simulink model "CM640C_MotAg1Meas"  (R2013b)
settings: Solver=VariableStepDiscrete  SolverMode=SingleTasking  StartTime=0.0  StopTime=1  FixedStep=0.002  RelTol=1e-3
values from neighbouring files (symbols this model uses):
  ARCHGLBPRM_2PI_ULS_F32 = DataDict.Constant    [CM640C_MotAg1Meas_DataDict.m]
  CNTPERREV_MOTREV_S15P16 = DataDict.Constant    [CM640C_MotAg1Meas_DataDict.m]
  COEFFTBLELMSIZE_CNT_U08 = DataDict.Constant    [CM640C_MotAg1Meas_DataDict.m]
  COEFFTBLSIZE_CNT_U08 = DataDict.Constant    [CM640C_MotAg1Meas_DataDict.m]
  CORRNTBLAGSTEPSIZE_MATRAD_F32 = DataDict.Constant    [CM640C_MotAg1Meas_DataDict.m]
  CORRNTBLSIDXOFFS_CNT_U16 = DataDict.Constant    [CM640C_MotAg1Meas_DataDict.m]
  CORRNTBLSIZE_CNT_U16 = DataDict.Constant    [CM640C_MotAg1Meas_DataDict.m]
  CORRNTBLSIZEMASK_CNT_U08 = DataDict.Constant    [CM640C_MotAg1Meas_DataDict.m]
  MOTAG1ERRTHD_MOTREV_U0P16 = DataDict.Constant    [CM640C_MotAg1Meas_DataDict.m]
  MotAg1MeasMotAgOffs = DataDict.Calibration    [CM640C_MotAg1Meas_DataDict.m]
  MotAg1PrtclFlt = DataDict.NTC    [CM640C_MotAg1Meas_DataDict.m]
  MOTAG1PRTCLFLTFAILSTEP_CNT_U16 = DataDict.Constant    [CM640C_MotAg1Meas_DataDict.m]
  MOTAG1PRTCLFLTPASSSTEP_CNT_U16 = DataDict.Constant    [CM640C_MotAg1Meas_DataDict.m]
  MOTAGCPTLIMFLTMASK_CNT_U32 = DataDict.Constant    [CM640C_MotAg1Meas_DataDict.m]
  MOTAGDELTAPERCORRNPT_CNT_U16 = DataDict.Constant    [CM640C_MotAg1Meas_DataDict.m]
  MOTAGFLTMASK_CNT_U32 = DataDict.Constant    [CM640C_MotAg1Meas_DataDict.m]
  MOTAGIDXMASK_CNT_U16 = DataDict.Constant    [CM640C_MotAg1Meas_DataDict.m]
  MOTAGLIMMASK_CNT_S32 = DataDict.Constant    [CM640C_MotAg1Meas_DataDict.m]
  MOTAGMGNLIMFLTMASK_CNT_U32 = DataDict.Constant    [CM640C_MotAg1Meas_DataDict.m]
  MOTAGMINWAITPERD_CNT_U32 = DataDict.Constant    [CM640C_MotAg1Meas_DataDict.m]
  MOTAGOFFS_CNT_S32 = DataDict.Constant    [CM640C_MotAg1Meas_DataDict.m]
  MOTAGOVFFLTMASK_CNT_U32 = DataDict.Constant    [CM640C_MotAg1Meas_DataDict.m]
  MOTAGSPITRSMMASK_CNT_U32 = DataDict.Constant    [CM640C_MotAg1Meas_DataDict.m]
  MOTAGVLTGFLTMASK_CNT_U32 = DataDict.Constant    [CM640C_MotAg1Meas_DataDict.m]
  NOMOTAGFLTMASK_CNT_U32 = DataDict.Constant    [CM640C_MotAg1Meas_DataDict.m]
  READBUFADR_CNT_U32 = DataDict.Constant    [CM640C_MotAg1Meas_DataDict.m]
  READBUFIDX_CNT_U08 = DataDict.Constant    [CM640C_MotAg1Meas_DataDict.m]
  SNSRAGMASK_CNT_U32 = DataDict.Constant    [CM640C_MotAg1Meas_DataDict.m]
  SNSRCNTMASK_CNT_U32 = DataDict.Constant    [CM640C_MotAg1Meas_DataDict.m]
  SPIAGCNTREGIDX_CNT_U08 = DataDict.Constant    [CM640C_MotAg1Meas_DataDict.m]
  SPIAGREGIDX_CNT_U08 = DataDict.Constant    [CM640C_MotAg1Meas_DataDict.m]
  SPISTATREGIDX_CNT_U08 = DataDict.Constant    [CM640C_MotAg1Meas_DataDict.m]
  SPITURNCNTRREGIDX_CNT_U08 = DataDict.Constant    [CM640C_MotAg1Meas_DataDict.m]
  STRTPTRINITVAL_CNT_U32 = DataDict.Constant    [CM640C_MotAg1Meas_DataDict.m]
  STRTPTRPERVAL_CNT_U32 = DataDict.Constant    [CM640C_MotAg1Meas_DataDict.m]
  TURNCNTRHALFOFFS_CNT_S16 = DataDict.Constant    [CM640C_MotAg1Meas_DataDict.m]
  TURNCNTROFFS_CNT_S16 = DataDict.Constant    [CM640C_MotAg1Meas_DataDict.m]
  TURNCNTRREGMASK_CNT_U32 = DataDict.Constant    [CM640C_MotAg1Meas_DataDict.m]
  VLDMOTAGFLTMASK_CNT_U32 = DataDict.Constant    [CM640C_MotAg1Meas_DataDict.m]
undefined symbols (not defined in the file or in its folder): NtcSts1, sigbuilder_block
libraries: simulink x41, FloatToFixd x1, NxtrMax x1
(part 3 of 7)

== system CM640C_MotAg1Meas/MotAg1Meas/MotAg1MeasPer2/MotAg1Calcn/MotAg1Processing/Offset Compensation  ==
  MotAg4Mecl : Inport  RequirementInfo={} %GIDa_25aaecee_4f2e_400f_abc5_f2372d041e99
  MotAg1SpiMecl : Inport  RequirementInfo={} %GIDa_27418f5d_8a5b_4847_ba52_ca2cb341472d  Port=2
  CopyRight2 : Subsystem  Description=|  mask(Copyright Information){none=on}
      | Copyright info block.                                               
      |                                                                     
      | Place copyright information at the top of every subsystem in design.
      mask prompts: none "No parameters"
      mask help: Place copyright information at the top of every subsystem in design.
      mask Display:
      | NxtrConf = 'Nexteer Confidential';
      | 
      | sys = bdroot; %handle for the current model ("system")
      | first = get_param(sys,'Created');
      | first = first(end-3:end);  %year is last four digits
      | 
      | last = get_param(sys,'LastModifiedDate');
      | if isempty(last)
      |     last = datestr(now,'yyyy');
      | else
      |     last = last(end-3:end);
      | end
      | 
      | if strcmp(first,last)
      |     fprintf('%s -- Copyright %s Nexteer',NxtrConf,first)
      | else
      |     fprintf('%s -- %s%s- %s Nexteer',NxtrConf,char(169),first,last)
      | end
  Data Store Read : DataStoreRead  DataStoreName=MotAg1InitOffs
  Data Store Write : DataStoreWrite  DataStoreName=MotAg1PrevOffs
  Data Store Write1 : DataStoreWrite  DataStoreName=dMotAg1MeasMotAg1RtOffs
  First Time Offset Calcn : Subsystem
  If : If  IfExpression=u1==0
  Merge : Merge
  Rt Offs Calcn : Subsystem
  Scope : Scope  NumInputPorts=2
      settings: AttributesFormatString=Simulation Only  YMin=0~0  YMax=17000~70000  SaveName=ScopeData2
  MotAg1Offs : Outport
  wires:
  MotAg1SpiMecl/1 -> First Time Offset Calcn/2(MotAg1SpiMecl), Rt Offs Calcn/2(MotAg1SpiMecl)
  Data Store Read/1 -> If/1
  If/1 -> First Time Offset Calcn/Action
  If/2 -> Rt Offs Calcn/Action
  Rt Offs Calcn/2(MotAg1RtOffs) -> Scope/2, Data Store Write1/1
  First Time Offset Calcn/1(MotAg1Offs) -> Merge/1
  Rt Offs Calcn/1(MotAg1Offs) -> Merge/2
  Merge/1 -> Data Store Write/1, Scope/1, MotAg1Offs/1
  MotAg4Mecl/1 -> Rt Offs Calcn/1(MotAg4Mecl), First Time Offset Calcn/1(MotAg4Mecl)

== system CM640C_MotAg1Meas/MotAg1Meas/MotAg1MeasPer2/MotAg1Calcn/MotAg1Processing/SPI  Motor Angle Calcn ==
  MotAg1RawReg : Inport
  MotAgMecl1Polarity : Inport  Port=2
  15-bit Angle Val : simulink/Logic and Bit Operations/Bitwise Operator  logicop=AND  UseBitMask=off  NumInputPorts=2  BitMask=SNSRVLTGFLTMASK_CNT_U32  BitMaskRealWorld=Stored Integer
  32767 : Constant  Value=SNSRAGMASK_CNT_U32
  AVAL Register : LookupNDDirect  NumberOfTableDimensions=1  TableIsInput=on
  Constant5 : Constant  Value=SPIAGREGIDX_CNT_U08
  Convert to p16 : ArithShift  BitShiftNumber=1  BitShiftDirection=Left
  CopyRight1 : Subsystem  Description=|  mask(Copyright Information){none=on}
      | Copyright info block.                                               
      |                                                                     
      | Place copyright information at the top of every subsystem in design.
      mask prompts: none "No parameters"
      mask help: Place copyright information at the top of every subsystem in design.
      mask Display:
      | NxtrConf = 'Nexteer Confidential';
      | 
      | sys = bdroot; %handle for the current model ("system")
      | first = get_param(sys,'Created');
      | first = first(end-3:end);  %year is last four digits
      | 
      | last = get_param(sys,'LastModifiedDate');
      | if isempty(last)
      |     last = datestr(now,'yyyy');
      | else
      |     last = last(end-3:end);
      | end
      | 
      | if strcmp(first,last)
      |     fprintf('%s -- Copyright %s Nexteer',NxtrConf,first)
      | else
      |     fprintf('%s -- %s%s- %s Nexteer',NxtrConf,char(169),first,last)
      | end
  Data Type Conversion1 : DataTypeConversion  OutDataTypeStr=uint16
  Display Variable1 : DataStoreWrite  DataStoreName=dMotAg1MeasMotAg1RawAgReg
  Polarity Correction : Subsystem  RequirementInfo="{'linktype_rmi_doors' '00011b54 (/ESG Group/FDD Module Requirements/EA4 Specific/CM640C_MotAg1Meas)' '#CM640C_108' 'true' 'REQ:  CM640C_108' '' } %GIDa_2ccc2f51_8829_4d0a_b712_e30842e2cdc8"
  MotAg1SpiMecl : Outport
  wires:
  32767/1 -> 15-bit Angle Val/2
  15-bit Angle Val/1 -> Data Type Conversion1/1
  Constant5/1 -> AVAL Register/1
  AVAL Register/1 -> Display Variable1/1, 15-bit Angle Val/1
  MotAg1RawReg/1 -> AVAL Register/2
  Convert to p16/1 -> Polarity Correction/1(MotAg1RawSpiMecl)
  MotAgMecl1Polarity/1 -> Polarity Correction/2(MotAgMecl1Polarity)
  Polarity Correction/1(MotAg1SpiMecl) -> MotAg1SpiMecl/1
  Data Type Conversion1/1 -> Convert to p16/1

== system CM640C_MotAg1Meas/MotAg1Meas/MotAg1MeasPer2/MotAg1Calcn/MotAg1Processing/SPI IIF Motor Angle ==
  MotAg1RawRes : Inport  RequirementInfo={} %GIDa_0615be2d_aadc_4d1d_9c12_95199cb19787
  Constant1 : Constant  Value=SPIAGCNTREGIDX_CNT_U08
  CopyRight2 : Subsystem  Description=|  mask(Copyright Information){none=on}
      | Copyright info block.                                               
      |                                                                     
      | Place copyright information at the top of every subsystem in design.
      mask prompts: none "No parameters"
      mask help: Place copyright information at the top of every subsystem in design.
      mask Display:
      | NxtrConf = 'Nexteer Confidential';
      | 
      | sys = bdroot; %handle for the current model ("system")
      | first = get_param(sys,'Created');
      | first = first(end-3:end);  %year is last four digits
      | 
      | last = get_param(sys,'LastModifiedDate');
      | if isempty(last)
      |     last = datestr(now,'yyyy');
      | else
      |     last = last(end-3:end);
      | end
      | 
      | if strcmp(first,last)
      |     fprintf('%s -- Copyright %s Nexteer',NxtrConf,first)
      | else
      |     fprintf('%s -- %s%s- %s Nexteer',NxtrConf,char(169),first,last)
      | end
  Data Store Write2 : DataStoreWrite  DataStoreName=dMotAg1MeasMotAg1SpiCntrAg
  IIF Count Register : LookupNDDirect  NumberOfTableDimensions=1  TableIsInput=on
  SpiMotAgCnt : Subsystem
  wires:
  MotAg1RawRes/1 -> IIF Count Register/2
  Constant1/1 -> IIF Count Register/1
  IIF Count Register/1 -> SpiMotAgCnt/1(MotAg1AgCntReg)
  SpiMotAgCnt/1(MotAg1SpiCntr) -> Data Store Write2/1

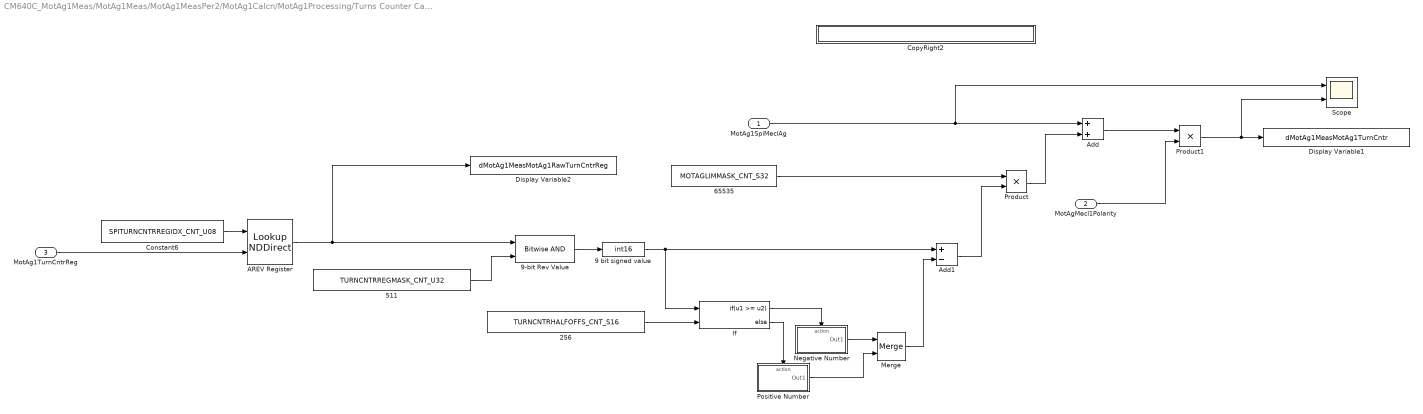
== system CM640C_MotAg1Meas/MotAg1Meas/MotAg1MeasPer2/MotAg1Calcn/MotAg1Processing/Turns Counter Calcn ==
  MotAg1SpiMeclAg : Inport
  MotAgMecl1Polarity : Inport  Port=2
  MotAg1TurnCntrReg : Inport  Port=3
  256 : Constant  Value=TURNCNTRHALFOFFS_CNT_S16
  511 : Constant  Value=TURNCNTRREGMASK_CNT_U32
  65535 : Constant  Value=MOTAGLIMMASK_CNT_S32
  9 bit signed value : DataTypeConversion  OutDataTypeStr=int16
  9-bit Rev Value : simulink/Logic and Bit Operations/Bitwise Operator  logicop=AND  UseBitMask=off  NumInputPorts=2  BitMask=SNSRVLTGFLTMASK_CNT_U32  BitMaskRealWorld=Stored Integer
  AREV Register : LookupNDDirect  NumberOfTableDimensions=1  TableIsInput=on
  Add : Sum
  Add1 : Sum  Inputs=+-
  Constant6 : Constant  Value=SPITURNCNTRREGIDX_CNT_U08  OutDataTypeStr=single
  CopyRight2 : Subsystem  Description=|  mask(Copyright Information){none=on}
      | Copyright info block.                                               
      |                                                                     
      | Place copyright information at the top of every subsystem in design.
      mask prompts: none "No parameters"
      mask help: Place copyright information at the top of every subsystem in design.
      mask Display:
      | NxtrConf = 'Nexteer Confidential';
      | 
      | sys = bdroot; %handle for the current model ("system")
      | first = get_param(sys,'Created');
      | first = first(end-3:end);  %year is last four digits
      | 
      | last = get_param(sys,'LastModifiedDate');
      | if isempty(last)
      |     last = datestr(now,'yyyy');
      | else
      |     last = last(end-3:end);
      | end
      | 
      | if strcmp(first,last)
      |     fprintf('%s -- Copyright %s Nexteer',NxtrConf,first)
      | else
      |     fprintf('%s -- %s%s- %s Nexteer',NxtrConf,char(169),first,last)
      | end
  Display Variable1 : DataStoreWrite  DataStoreName=dMotAg1MeasMotAg1TurnCntr
  Display Variable2 : DataStoreWrite  DataStoreName=dMotAg1MeasMotAg1RawTurnCntrReg
  If : If  RequirementInfo={} %GIDa_1dcda5a9_5c02_4c7c_90a0_60f3e0279390  NumInputs=2  IfExpression=u1 >= u2
  Merge : Merge
  Negative Number : Subsystem  RequirementInfo={} %GIDa_ef2e3230_8676_4b3c_b77c_df6f21b77702  TreatAsAtomicUnit=on
  Positive Number : Subsystem  RequirementInfo={} %GIDa_540b1f9f_51f9_4273_8cc8_b201940ca857  TreatAsAtomicUnit=on
  Product : Product
  Product1 : Product  OutDataTypeStr=single
  Scope : Scope  NumInputPorts=2
      settings: AttributesFormatString=Simulation Only  YMin=0~0  YMax=17000~70000  SaveName=ScopeData8
  wires:
  511/1 -> 9-bit Rev Value/2
  65535/1 -> Product/1
  Product/1 -> Add/2
  Add/1 -> Product1/1
  Product1/1 -> Scope/2, Display Variable1/1
  9 bit signed value/1 -> Add1/1, If/1
  If/1 -> Negative Number/Action
  If/2 -> Positive Number/Action
  Negative Number/1(Out1) -> Merge/1
  Positive Number/1(Out1) -> Merge/2
  Merge/1 -> Add1/2
  256/1 -> If/2
  Constant6/1 -> AREV Register/1
  MotAg1TurnCntrReg/1 -> AREV Register/2
  AREV Register/1 -> Display Variable2/1, 9-bit Rev Value/1
  MotAgMecl1Polarity/1 -> Product1/2
  MotAg1SpiMeclAg/1 -> Scope/1, Add/1
  Add1/1 -> Product/2
  9-bit Rev Value/1 -> 9 bit signed value/1

== system CM640C_MotAg1Meas/MotAg1Meas/MotAg1MeasPer2/MotAg1Calcn/SpiRx/CopyRight2 ==

== system CM640C_MotAg1Meas/MotAg1Meas/MotAg1MeasPer2/MotAg1Calcn/SpiRx/Data ==
  note: Code Ref:
      | MotAg1RawRegBuf_Cnt_u32[SpiReadCntr_Cnt_T_u08] = CSIH3RX0W;
      | dPimMotAg1RawReg[SpiReadCntr_Cnt_T_u08] = MotAg1RawRegBuf_Cnt_u32[SpiReadCntr_Cnt_T_u08];
  note: Register Read
      | Defined as Inp
  note: Follow below steps in same order:
      |
      | 1. Read from the register RegInptCSIH3RX0W.(Start address is mentioned, Address is incremented).
      | 2. For every increment of the address, new value is obtained in Register.
      | 3. Assign it to a local variable as an array.
  note: Note: Read the Register only once in the for loop. use a local variable and add it to the display variable
  N : Inport
  Assignment : Assignment  IndexMode=Zero-based  OutputInitialize=Specify size for each dimension in table  IndexOptions=Index vector (port)  Indices=[17]  OutputSizes=10
  CopyRight2 : Subsystem  Description=|  mask(Copyright Information){none=on}
      | Copyright info block.                                               
      |                                                                     
      | Place copyright information at the top of every subsystem in design.
      mask prompts: none "No parameters"
      mask help: Place copyright information at the top of every subsystem in design.
      mask Display:
      | NxtrConf = 'Nexteer Confidential';
      | 
      | sys = bdroot; %handle for the current model ("system")
      | first = get_param(sys,'Created');
      | first = first(end-3:end);  %year is last four digits
      | 
      | last = get_param(sys,'LastModifiedDate');
      | if isempty(last)
      |     last = datestr(now,'yyyy');
      | else
      |     last = last(end-3:end);
      | end
      | 
      | if strcmp(first,last)
      |     fprintf('%s -- Copyright %s Nexteer',NxtrConf,first)
      | else
      |     fprintf('%s -- %s%s- %s Nexteer',NxtrConf,char(169),first,last)
      | end
  Data Store Write : DataStoreWrite  DataStoreName=dMotAg1MeasMotAg1RawReg
  For Iterator : ForIterator  IterationSource=external  IterationLimit=7  IndexMode=Zero-based
  RegInptCSIH3RX0W : Ground
  Selector : Selector  IndexMode=Zero-based  InputPortWidth=10  IndexOptions=Index vector (port)  Indices=[1 3]  OutputSizes=1
  Simulation Only : DataStoreRead  DataStoreName=RxBuffer
  Terminator : Terminator
  MotAg1RawRegBuf : Outport
  wires:
  Selector/1 -> Assignment/1
  For Iterator/1 -> Selector/2, Assignment/2
  Simulation Only/1 -> Selector/1
  N/1 -> For Iterator/1
  RegInptCSIH3RX0W/1 -> Terminator/1
  Assignment/1 -> MotAg1RawRegBuf/1, Data Store Write/1

== system CM640C_MotAg1Meas/MotAg1Meas/MotAg1MeasPer3/Initial Check/IdleState SendTx/CopyRight2 ==

== system CM640C_MotAg1Meas/MotAg1Meas/MotAg1MeasPer3/Initial Check/IdleState SendTx/Flt Cntr Ena ==
  CopyRight2 : Subsystem  Description=|  mask(Copyright Information){none=on}
      | Copyright info block.                                               
      |                                                                     
      | Place copyright information at the top of every subsystem in design.
      mask prompts: none "No parameters"
      mask help: Place copyright information at the top of every subsystem in design.
      mask Display:
      | NxtrConf = 'Nexteer Confidential';
      | 
      | sys = bdroot; %handle for the current model ("system")
      | first = get_param(sys,'Created');
      | first = first(end-3:end);  %year is last four digits
      | 
      | last = get_param(sys,'LastModifiedDate');
      | if isempty(last)
      |     last = datestr(now,'yyyy');
      | else
      |     last = last(end-3:end);
      | end
      | 
      | if strcmp(first,last)
      |     fprintf('%s -- Copyright %s Nexteer',NxtrConf,first)
      | else
      |     fprintf('%s -- %s%s- %s Nexteer',NxtrConf,char(169),first,last)
      | end
  Data Store Read : DataStoreRead  DataStoreName=MotAg1PrevSpiErrFltCntr
  If : If  IfExpression=u1==65535
  Merge : Merge
  Wrap back to 0 : Subsystem  TreatAsAtomicUnit=on
  i++ : Subsystem  TreatAsAtomicUnit=on
  MotAg1SpiTrsmFltCntr : Outport
  wires:
  Data Store Read/1 -> If/1
  If/1 -> Wrap back to 0/Action
  If/2 -> i++/Action
  Wrap back to 0/1(MotAg1SpiTrsmFltCntr) -> Merge/1
  i++/1(MotAg1SpiTrsmFltCntr) -> Merge/2
  Merge/1 -> MotAg1SpiTrsmFltCntr/1

== system CM640C_MotAg1Meas/MotAg1Meas/MotAg1MeasPer3/Initial Check/IdleState SendTx/MotAg1Sync ==
  note: Follow below steps in same order:
      |
      | 1. Set Chip Select PIN of CSIH3 peripheral to GPIO mode. (PIN as output).
      | 2. Set Chip Select of CSIH3 to Low.
      | 3. Get System time and run it once. Run the TiSpan until it is = 2 microsecond
      | 4. Set Chip Select of CSIH3 to High.
      | 5. Get MotAg4 (ENCA Interface Aggle to synchronize with SPI Angle).
      | 6. Map back the Chip Select PIN back to CSIH peripheral mode.
      | 7. Transmit Tx messeges.
      | 8. Read IIF angle (from motor control loop, PIM)
  CopyRight2 : Subsystem  Description=|  mask(Copyright Information){none=on}
      | Copyright info block.                                               
      |                                                                     
      | Place copyright information at the top of every subsystem in design.
      mask prompts: none "No parameters"
      mask help: Place copyright information at the top of every subsystem in design.
      mask Display:
      | NxtrConf = 'Nexteer Confidential';
      | 
      | sys = bdroot; %handle for the current model ("system")
      | first = get_param(sys,'Created');
      | first = first(end-3:end);  %year is last four digits
      | 
      | last = get_param(sys,'LastModifiedDate');
      | if isempty(last)
      |     last = datestr(now,'yyyy');
      | else
      |     last = last(end-3:end);
      | end
      | 
      | if strcmp(first,last)
      |     fprintf('%s -- Copyright %s Nexteer',NxtrConf,first)
      | else
      |     fprintf('%s -- %s%s- %s Nexteer',NxtrConf,char(169),first,last)
      | end
  Data Store Read : DataStoreRead  Priority=80  DataStoreName=MotAg1Diagc
  GetMotAg4Mecl : Subsystem  RequirementInfo={} %GIDa_e9ea58e3_6a41_40f8_8e21_748bdef8f324  Priority=50
      settings: AttributesFormatString=Priority = %<Priority>
  IoHwAb_SetFctGpioMotAg1 : Subsystem  RequirementInfo={} %GIDa_22c35125_a8ba_4460_94b4_245c6f19b05d  Priority=10
      settings: AttributesFormatString=Priority = %<Priority>
  IoHwAb_SetFctPrphlMotAg1 : Subsystem  Priority=60
      settings: AttributesFormatString=Priority = %<Priority>
  Set Chip Select High : Subsystem  Priority=40
      settings: AttributesFormatString=Priority = %<Priority>
  Set Chip Select Low : Subsystem  Priority=20
      settings: AttributesFormatString=Priority = %<Priority>
  SpiTx : Subsystem  Priority=70
      settings: AttributesFormatString=Priority = %<Priority>
  Wait for 2us : Subsystem  Priority=30
      settings: AttributesFormatString=Priority = %<Priority>
  MotAg4Mecl : Outport
  MotAg1DiagcAg : Outport  Port=2
  wires:
  GetMotAg4Mecl/1(MotAg4Mecl) -> MotAg4Mecl/1
  Data Store Read/1 -> MotAg1DiagcAg/1

== system CM640C_MotAg1Meas/MotAg1Meas/MotAg1MeasPer3/Initial Check/InitTxCommunication going on Wait/CopyRight2 ==

== system CM640C_MotAg1Meas/MotAg1Meas/MotAg1MeasPer3/Initial Check/InitTxCommunication going on Wait/Last Flt Cntr  ==
  CopyRight2 : Subsystem  Description=|  mask(Copyright Information){none=on}
      | Copyright info block.                                               
      |                                                                     
      | Place copyright information at the top of every subsystem in design.
      mask prompts: none "No parameters"
      mask help: Place copyright information at the top of every subsystem in design.
      mask Display:
      | NxtrConf = 'Nexteer Confidential';
      | 
      | sys = bdroot; %handle for the current model ("system")
      | first = get_param(sys,'Created');
      | first = first(end-3:end);  %year is last four digits
      | 
      | last = get_param(sys,'LastModifiedDate');
      | if isempty(last)
      |     last = datestr(now,'yyyy');
      | else
      |     last = last(end-3:end);
      | end
      | 
      | if strcmp(first,last)
      |     fprintf('%s -- Copyright %s Nexteer',NxtrConf,first)
      | else
      |     fprintf('%s -- %s%s- %s Nexteer',NxtrConf,char(169),first,last)
      | end
  Data Store Read : DataStoreRead  DataStoreName=MotAg1PrevSpiErrFltCntr
  MotAg1SpiTrsmFltCntr : Outport
  wires:
  Data Store Read/1 -> MotAg1SpiTrsmFltCntr/1

== system CM640C_MotAg1Meas/Sensor Simulated Values/Signal Processing/Simulated Enca Angle/Subsystem/CopyRight2 ==

== system CM640C_MotAg1Meas/MotAg1Meas/MotAg1MeasInit1/Compute Correction Table/NVM NOK/Zero out correction table/CopyRight2 ==

== system CM640C_MotAg1Meas/MotAg1Meas/MotAg1MeasInit1/Compute Correction Table/NVM Ok/Calculate Correction Table/Build Wave ==
  Constant : Constant  Value=CORRNTBLSIZE_CNT_U16
  CopyRight2 : Subsystem  Description=|  mask(Copyright Information){none=on}
      | Copyright info block.                                               
      |                                                                     
      | Place copyright information at the top of every subsystem in design.
      mask prompts: none "No parameters"
      mask help: Place copyright information at the top of every subsystem in design.
      mask Display:
      | NxtrConf = 'Nexteer Confidential';
      | 
      | sys = bdroot; %handle for the current model ("system")
      | first = get_param(sys,'Created');
      | first = first(end-3:end);  %year is last four digits
      | 
      | last = get_param(sys,'LastModifiedDate');
      | if isempty(last)
      |     last = datestr(now,'yyyy');
      | else
      |     last = last(end-3:end);
      | end
      | 
      | if strcmp(first,last)
      |     fprintf('%s -- Copyright %s Nexteer',NxtrConf,first)
      | else
      |     fprintf('%s -- %s%s- %s Nexteer',NxtrConf,char(169),first,last)
      | end
  Reconstructed Waveform Processing : Subsystem  TreatAsAtomicUnit=on
  wires:
  Constant/1 -> Reconstructed Waveform Processing/1(N)

== system CM640C_MotAg1Meas/MotAg1Meas/MotAg1MeasInit1/Compute Correction Table/NVM Ok/Calculate Correction Table/Change Correction Coordinate ==
  Constant1 : Constant  Value=CORRNTBLSIZE_CNT_U16
  CopyRight2 : Subsystem  Description=|  mask(Copyright Information){none=on}
      | Copyright info block.                                               
      |                                                                     
      | Place copyright information at the top of every subsystem in design.
      mask prompts: none "No parameters"
      mask help: Place copyright information at the top of every subsystem in design.
      mask Display:
      | NxtrConf = 'Nexteer Confidential';
      | 
      | sys = bdroot; %handle for the current model ("system")
      | first = get_param(sys,'Created');
      | first = first(end-3:end);  %year is last four digits
      | 
      | last = get_param(sys,'LastModifiedDate');
      | if isempty(last)
      |     last = datestr(now,'yyyy');
      | else
      |     last = last(end-3:end);
      | end
      | 
      | if strcmp(first,last)
      |     fprintf('%s -- Copyright %s Nexteer',NxtrConf,first)
      | else
      |     fprintf('%s -- %s%s- %s Nexteer',NxtrConf,char(169),first,last)
      | end
  Waveform Coordinate Change : Subsystem  TreatAsAtomicUnit=on
  wires:
  Constant1/1 -> Waveform Coordinate Change/1(N)

== system CM640C_MotAg1Meas/MotAg1Meas/MotAg1MeasInit1/Compute Correction Table/NVM Ok/Calculate Correction Table/CopyRight2 ==

== system CM640C_MotAg1Meas/MotAg1Meas/MotAg1MeasInit1/Compute Correction Table/NVM Ok/Configure Coefficients/CopyRight2 ==

== system CM640C_MotAg1Meas/MotAg1Meas/MotAg1MeasPer1/Motor Angle Processing/Offset /Compensate MechMotPos/CopyRight2 ==

== system CM640C_MotAg1Meas/MotAg1Meas/MotAg1MeasPer2/MotAg1Calcn/MotAg1Processing/Diagnostics/ Qualifier Sts ==
  note: Function Call Sequence Requirements
      |
      | - GetNtcQlfr shall execute after SetNtcSts
  NtcStInfo : Inport
  Constant3 : Constant  Value=MotAg1PrtclFlt
  CopyRight2 : Subsystem  Description=|  mask(Copyright Information){none=on}
      | Copyright info block.                                               
      |                                                                     
      | Place copyright information at the top of every subsystem in design.
      mask prompts: none "No parameters"
      mask help: Place copyright information at the top of every subsystem in design.
      mask Display:
      | NxtrConf = 'Nexteer Confidential';
      | 
      | sys = bdroot; %handle for the current model ("system")
      | first = get_param(sys,'Created');
      | first = first(end-3:end);  %year is last four digits
      | 
      | last = get_param(sys,'LastModifiedDate');
      | if isempty(last)
      |     last = datestr(now,'yyyy');
      | else
      |     last = last(end-3:end);
      | end
      | 
      | if strcmp(first,last)
      |     fprintf('%s -- Copyright %s Nexteer',NxtrConf,first)
      | else
      |     fprintf('%s -- %s%s- %s Nexteer',NxtrConf,char(169),first,last)
      | end
  GetNtcQlfr : Subsystem  RequirementInfo={} %GIDa_b7a1ef15_bb0a_401a_885b_7c93fc316d4b
  NtcSts and DebStep Calcn : Subsystem  TreatAsAtomicUnit=on
  Scope1 : Scope
      settings: RequirementInfo={} %GIDa_e81b7e69_0b94_4617_9cae_9ecdf9c9f643  SaveName=ScopeData19
  SetNtcSts : Subsystem  RequirementInfo={} %GIDa_cc16d2b9_ba62_49e4_845a_b1ea47e91fec
  U8 to Enum : DataTypeConversion  OutDataTypeStr=Enum: SigQlfr1
  MotAg1MeclQlfr : Outport  RequirementInfo={} %GIDa_fa47d6bf_629d_438f_b5f4_d3c79a485692
  wires:
  NtcStInfo/1 -> SetNtcSts/2(NtcStInfo), NtcSts and DebStep Calcn/1(NtcStInfo)
  Constant3/1 -> SetNtcSts/1(NtcNr), GetNtcQlfr/1(NtcNr)  "NtcNr"
  GetNtcQlfr/1(NtcQlfr) -> U8 to Enum/1
  NtcSts and DebStep Calcn/1(NtcSts) -> SetNtcSts/3(NtcSts)
  NtcSts and DebStep Calcn/2(DebStep) -> SetNtcSts/4(DebStep), Scope1/1
  U8 to Enum/1 -> MotAg1MeclQlfr/1

== system CM640C_MotAg1Meas/MotAg1Meas/MotAg1MeasPer2/MotAg1Calcn/MotAg1Processing/Diagnostics/CopyRight2 ==

== system CM640C_MotAg1Meas/MotAg1Meas/MotAg1MeasPer2/MotAg1Calcn/MotAg1Processing/Diagnostics/Offset = 0 ==
  Action Port : ActionPort  ActionType=else
  Constant3 : Constant  Value=0  OutDataTypeStr=int32
  CopyRight2 : Subsystem  Description=|  mask(Copyright Information){none=on}
      | Copyright info block.                                               
      |                                                                     
      | Place copyright information at the top of every subsystem in design.
      mask prompts: none "No parameters"
      mask help: Place copyright information at the top of every subsystem in design.
      mask Display:
      | NxtrConf = 'Nexteer Confidential';
      | 
      | sys = bdroot; %handle for the current model ("system")
      | first = get_param(sys,'Created');
      | first = first(end-3:end);  %year is last four digits
      | 
      | last = get_param(sys,'LastModifiedDate');
      | if isempty(last)
      |     last = datestr(now,'yyyy');
      | else
      |     last = last(end-3:end);
      | end
      | 
      | if strcmp(first,last)
      |     fprintf('%s -- Copyright %s Nexteer',NxtrConf,first)
      | else
      |     fprintf('%s -- %s%s- %s Nexteer',NxtrConf,char(169),first,last)
      | end
  Offset : Outport
  wires:
  Constant3/1 -> Offset/1

== system CM640C_MotAg1Meas/MotAg1Meas/MotAg1MeasPer2/MotAg1Calcn/MotAg1Processing/Diagnostics/Offset = 1 ==
  Action Port : ActionPort  ActionType=then
  Constant3 : Constant  Value=CNTPERREV_MOTREV_S15P16
  CopyRight2 : Subsystem  Description=|  mask(Copyright Information){none=on}
      | Copyright info block.                                               
      |                                                                     
      | Place copyright information at the top of every subsystem in design.
      mask prompts: none "No parameters"
      mask help: Place copyright information at the top of every subsystem in design.
      mask Display:
      | NxtrConf = 'Nexteer Confidential';
      | 
      | sys = bdroot; %handle for the current model ("system")
      | first = get_param(sys,'Created');
      | first = first(end-3:end);  %year is last four digits
      | 
      | last = get_param(sys,'LastModifiedDate');
      | if isempty(last)
      |     last = datestr(now,'yyyy');
      | else
      |     last = last(end-3:end);
      | end
      | 
      | if strcmp(first,last)
      |     fprintf('%s -- Copyright %s Nexteer',NxtrConf,first)
      | else
      |     fprintf('%s -- %s%s- %s Nexteer',NxtrConf,char(169),first,last)
      | end
  Offset : Outport
  wires:
  Constant3/1 -> Offset/1

== system CM640C_MotAg1Meas/MotAg1Meas/MotAg1MeasPer2/MotAg1Calcn/MotAg1Processing/Diagnostics/Rolling Counter ==
  Test_Lgc : Inport
  CopyRight2 : Subsystem  Description=|  mask(Copyright Information){none=on}
      | Copyright info block.                                               
      |                                                                     
      | Place copyright information at the top of every subsystem in design.
      mask prompts: none "No parameters"
      mask help: Place copyright information at the top of every subsystem in design.
      mask Display:
      | NxtrConf = 'Nexteer Confidential';
      | 
      | sys = bdroot; %handle for the current model ("system")
      | first = get_param(sys,'Created');
      | first = first(end-3:end);  %year is last four digits
      | 
      | last = get_param(sys,'LastModifiedDate');
      | if isempty(last)
      |     last = datestr(now,'yyyy');
      | else
      |     last = last(end-3:end);
      | end
      | 
      | if strcmp(first,last)
      |     fprintf('%s -- Copyright %s Nexteer',NxtrConf,first)
      | else
      |     fprintf('%s -- %s%s- %s Nexteer',NxtrConf,char(169),first,last)
      | end
  Data Store Write : DataStoreWrite  DataStoreName=MotAg1PrevRollgCntr
  If : If  IfExpression=u1==0
  Merge : Merge
  Test Faild : Subsystem  TreatAsAtomicUnit=on
  Test Pass : Subsystem  TreatAsAtomicUnit=on
  MotAg1MeclRollgCntr : Outport
  wires:
  Merge/1 -> MotAg1MeclRollgCntr/1, Data Store Write/1
  Test Faild/1(RollgCntr) -> Merge/2
  Test Pass/1(RollgCntr) -> Merge/1
  If/2 -> Test Faild/Action
  If/1 -> Test Pass/Action
  Test_Lgc/1 -> If/1

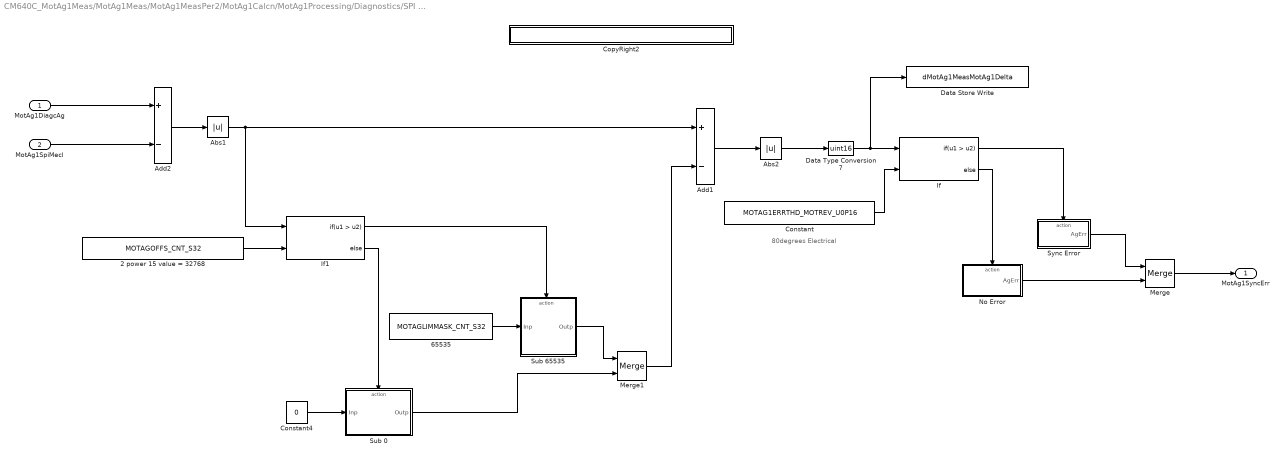
== system CM640C_MotAg1Meas/MotAg1Meas/MotAg1MeasPer2/MotAg1Calcn/MotAg1Processing/Diagnostics/SPI vs ENCA ==
  note: 80degrees Electrical
  MotAg1DiagcAg : Inport
  MotAg1SpiMecl : Inport  Port=2
  2 power 15 value = 32768 : Constant  Value=MOTAGOFFS_CNT_S32
  65535 : Constant  Value=MOTAGLIMMASK_CNT_S32
  Abs1 : Abs
  Abs2 : Abs
  Add1 : Sum  Inputs=+-  AccumDataTypeStr=int32
  Add2 : Sum  Inputs=+-  AccumDataTypeStr=int32
  Constant : Constant  Value=MOTAG1ERRTHD_MOTREV_U0P16
  Constant4 : Constant  Value=0  OutDataTypeStr=int32
  CopyRight2 : Subsystem  Description=|  mask(Copyright Information){none=on}
      | Copyright info block.                                               
      |                                                                     
      | Place copyright information at the top of every subsystem in design.
      mask prompts: none "No parameters"
      mask help: Place copyright information at the top of every subsystem in design.
      mask Display:
      | NxtrConf = 'Nexteer Confidential';
      | 
      | sys = bdroot; %handle for the current model ("system")
      | first = get_param(sys,'Created');
      | first = first(end-3:end);  %year is last four digits
      | 
      | last = get_param(sys,'LastModifiedDate');
      | if isempty(last)
      |     last = datestr(now,'yyyy');
      | else
      |     last = last(end-3:end);
      | end
      | 
      | if strcmp(first,last)
      |     fprintf('%s -- Copyright %s Nexteer',NxtrConf,first)
      | else
      |     fprintf('%s -- %s%s- %s Nexteer',NxtrConf,char(169),first,last)
      | end
  Data Store Write : DataStoreWrite  DataStoreName=dMotAg1MeasMotAg1Delta
  Data Type Conversion7 : DataTypeConversion  OutDataTypeStr=uint16
  If : If  RequirementInfo="{'linktype_rmi_doors' '00011b54 (/ESG Group/FDD Module Requirements/EA4 Specific/CM640C_MotAg1Meas)' '#CM640C_27' 'true' 'REQ:  CM640C_27' '' } %GIDa_3a1f876d_048a_4124_8b9b_10784d2bdcd3"  NumInputs=2  IfExpression=u1 > u2
  If1 : If  NumInputs=2  IfExpression=u1 > u2
  Merge : Merge
  Merge1 : Merge
  No Error : Subsystem  TreatAsAtomicUnit=on
  Sub 0 : Subsystem  TreatAsAtomicUnit=on
  Sub 65535 : Subsystem  TreatAsAtomicUnit=on
  Sync Error : Subsystem  TreatAsAtomicUnit=on
  MotAg1SyncErr : Outport  RequirementInfo="{'linktype_rmi_doors' '00011b54 (/ESG Group/FDD Module Requirements/EA4 Specific/CM640C_MotAg1Meas)' '#CM640C_27' 'true' 'REQ:  CM640C_27' '' } %GIDa_87b1ef67_c1dd_4e06_93a7_67cd4cfd2c9b"
  wires:
  Sync Error/1(AgErr) -> Merge/1
  If/2 -> No Error/Action
  If/1 -> Sync Error/Action
  Data Type Conversion7/1 -> Data Store Write/1, If/1
  No Error/1(AgErr) -> Merge/2
  Merge/1 -> MotAg1SyncErr/1
  MotAg1DiagcAg/1 -> Add2/1
  MotAg1SpiMecl/1 -> Add2/2
  Abs1/1 -> If1/1, Add1/1
  Add2/1 -> Abs1/1
  Abs2/1 -> Data Type Conversion7/1
  Constant/1 -> If/2
  If1/1 -> Sub 65535/Action
  If1/2 -> Sub 0/Action
  Constant4/1 -> Sub 0/1(Inp)
  Sub 65535/1(Outp) -> Merge1/1
  Sub 0/1(Outp) -> Merge1/2
  Merge1/1 -> Add1/2
  Add1/1 -> Abs2/1
  65535/1 -> Sub 65535/1(Inp)
  2 power 15 value = 32768/1 -> If1/2

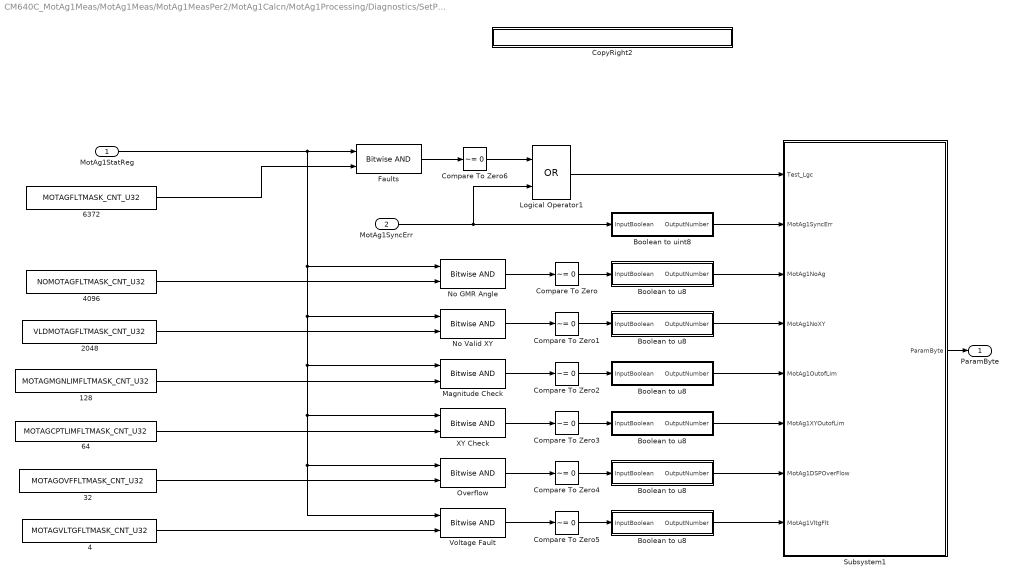
== system CM640C_MotAg1Meas/MotAg1Meas/MotAg1MeasPer2/MotAg1Calcn/MotAg1Processing/Diagnostics/SetParamByte ==
  MotAg1StatReg : Inport  RequirementInfo="{'linktype_rmi_doors' '00011b54 (/ESG Group/FDD Module Requirements/EA4 Specific/CM640C_MotAg1Meas)' '#CM640C_110' 'true' 'REQ:  CM640C_110' '' } %GIDa_ed1a1aae_91a4_4e1e_90c6_3e5d94cba6a2"
  MotAg1SyncErr : Inport  RequirementInfo={} %GIDa_e7e0662e_6f02_49f5_bf5b_7ffba48e0cf1  Port=2
  128 : Constant  RequirementInfo={} %GIDa_ee667166_d72d_44f1_9ab5_d6b4da4a8222  Value=MOTAGMGNLIMFLTMASK_CNT_U32  OutDataTypeStr=uint32
  2048 : Constant  RequirementInfo={} %GIDa_735b5020_5a5f_408c_9257_ab0056d227d2  Value=VLDMOTAGFLTMASK_CNT_U32  OutDataTypeStr=uint32
  32 : Constant  RequirementInfo={} %GIDa_5d33d96e_ca13_4b1c_8558_6c0ef8013d30  Value=MOTAGOVFFLTMASK_CNT_U32
  4 : Constant  RequirementInfo={} %GIDa_b4b00ad8_e272_4e38_b3ac_18dd32452033  Value=MOTAGVLTGFLTMASK_CNT_U32
  4096 : Constant  RequirementInfo={} %GIDa_bba271a7_4644_4e58_a214_f000267c6f8e  Value=NOMOTAGFLTMASK_CNT_U32
  6372 : Constant  RequirementInfo={} %GIDa_5e523a86_d58e_42f5_a3a2_01126440ea69  Value=MOTAGFLTMASK_CNT_U32
  64 : Constant  RequirementInfo={} %GIDa_3229e354_7906_42e2_b8f3_27f1ba396d7b  Value=MOTAGCPTLIMFLTMASK_CNT_U32
  Boolean to u8 : Subsystem  RequirementInfo={} %GIDa_2013d518_c891_4fcf_ac6f_a1ab1023bc8f  TreatAsAtomicUnit=on
  "Boolean to u8 " : Subsystem  RequirementInfo={} %GIDa_98ab4495_adb7_4b1b_b704_4d679a22b3b1  TreatAsAtomicUnit=on
  "Boolean to u8  " : Subsystem  RequirementInfo={} %GIDa_cf435d34_7987_416e_8f33_6373522ac39a  TreatAsAtomicUnit=on
  "Boolean to u8   " : Subsystem  RequirementInfo={} %GIDa_2d342136_aa03_46b1_a202_cbc6bdb78f26  TreatAsAtomicUnit=on
  "Boolean to u8    " : Subsystem  RequirementInfo={} %GIDa_3b4dff4f_1f82_402b_8bb5_7bcebcaf4f9e  TreatAsAtomicUnit=on
  "Boolean to u8     " : Subsystem  RequirementInfo={} %GIDa_f249d845_fe4e_48fe_b3af_b223b469c17e  TreatAsAtomicUnit=on
  Boolean to uint8 : Subsystem  RequirementInfo={} %GIDa_3a03cdd2_761e_466c_b322_4a3f4cbb014f  TreatAsAtomicUnit=on
  Compare To Zero : simulink/Logic and Bit Operations/Compare To Zero  RequirementInfo={} %GIDa_88f7f782_5d57_4e2e_870d_eb07d6a9c7ec  relop=~=  OutDataTypeStr=boolean
  Compare To Zero1 : simulink/Logic and Bit Operations/Compare To Zero  RequirementInfo={} %GIDa_06a8ec51_c8b9_4f29_b32c_6ed0bbf21673  relop=~=  OutDataTypeStr=boolean
  Compare To Zero2 : simulink/Logic and Bit Operations/Compare To Zero  RequirementInfo={} %GIDa_ee48c834_a1c4_4feb_9d87_859ad43caa65  relop=~=  OutDataTypeStr=boolean
  Compare To Zero3 : simulink/Logic and Bit Operations/Compare To Zero  RequirementInfo={} %GIDa_30cda4c8_6d55_46c6_9082_14f734000a42  relop=~=  OutDataTypeStr=boolean
  Compare To Zero4 : simulink/Logic and Bit Operations/Compare To Zero  RequirementInfo={} %GIDa_c96e8f21_4b08_4373_86af_051be6e61e42  relop=~=  OutDataTypeStr=boolean
  Compare To Zero5 : simulink/Logic and Bit Operations/Compare To Zero  RequirementInfo={} %GIDa_6186e4d8_cb6b_40d2_9714_9de370e63f5f  relop=~=  OutDataTypeStr=boolean
  Compare To Zero6 : simulink/Logic and Bit Operations/Compare To Zero  RequirementInfo={} %GIDa_1977373a_5a37_4741_9dc6_1734d289992d  relop=~=  OutDataTypeStr=boolean
  CopyRight2 : Subsystem  Description=|  mask(Copyright Information){none=on}
      | Copyright info block.                                               
      |                                                                     
      | Place copyright information at the top of every subsystem in design.
      mask prompts: none "No parameters"
      mask help: Place copyright information at the top of every subsystem in design.
      mask Display:
      | NxtrConf = 'Nexteer Confidential';
      | 
      | sys = bdroot; %handle for the current model ("system")
      | first = get_param(sys,'Created');
      | first = first(end-3:end);  %year is last four digits
      | 
      | last = get_param(sys,'LastModifiedDate');
      | if isempty(last)
      |     last = datestr(now,'yyyy');
      | else
      |     last = last(end-3:end);
      | end
      | 
      | if strcmp(first,last)
      |     fprintf('%s -- Copyright %s Nexteer',NxtrConf,first)
      | else
      |     fprintf('%s -- %s%s- %s Nexteer',NxtrConf,char(169),first,last)
      | end
  Faults : simulink/Logic and Bit Operations/Bitwise Operator  RequirementInfo={} %GIDa_27b0c683_c1dd_4260_8271_5f58b77987f5  logicop=AND  UseBitMask=off  NumInputPorts=2  BitMask=hex2dec('18E4')  BitMaskRealWorld=Stored Integer
  Logical Operator1 : Logic  RequirementInfo={} %GIDa_3b71d2af_c8c5_4605_a6fb_e86525b1f2bb  Operator=OR  AllPortsSameDT=off  OutDataTypeStr=boolean
  Magnitude Check : simulink/Logic and Bit Operations/Bitwise Operator  RequirementInfo={} %GIDa_e25437d7_a330_4cdd_b5c0_5b0161f572bd  logicop=AND  UseBitMask=off  NumInputPorts=2  BitMask=hex2dec('0080')  BitMaskRealWorld=Stored Integer
  No GMR Angle : simulink/Logic and Bit Operations/Bitwise Operator  RequirementInfo={} %GIDa_62a9aad4_017d_4660_bed6_fb7fd858f242  logicop=AND  UseBitMask=off  NumInputPorts=2  BitMask=hex2dec('1000')  BitMaskRealWorld=Stored Integer
  No Valid XY : simulink/Logic and Bit Operations/Bitwise Operator  RequirementInfo={} %GIDa_cdc42c7a_e72d_4adc_859a_bcf854984fec  logicop=AND  UseBitMask=off  NumInputPorts=2  BitMask=hex2dec('0800')  BitMaskRealWorld=Stored Integer
  Overflow : simulink/Logic and Bit Operations/Bitwise Operator  RequirementInfo={} %GIDa_cd6df461_a107_4156_bc5d_3340ec7e0b34  logicop=AND  UseBitMask=off  NumInputPorts=2  BitMask=hex2dec('0020')  BitMaskRealWorld=Stored Integer
  Subsystem1 : Subsystem  RequirementInfo={} %GIDa_2d88dca2_c0ec_4920_869b_cee079956af9
  Voltage Fault : simulink/Logic and Bit Operations/Bitwise Operator  RequirementInfo={} %GIDa_95b6da90_17d3_447e_a2b9_71565d701bd0  logicop=AND  UseBitMask=off  NumInputPorts=2  BitMask=hex2dec('0004')  BitMaskRealWorld=Stored Integer
  XY Check : simulink/Logic and Bit Operations/Bitwise Operator  RequirementInfo={} %GIDa_1be1c5b2_1ea6_4c54_8d0f_5a568548fcca  logicop=AND  UseBitMask=off  NumInputPorts=2  BitMask=hex2dec('0040')  BitMaskRealWorld=Stored Integer
  ParamByte : Outport
  wires:
  4096/1 -> No GMR Angle/2
  2048/1 -> No Valid XY/2
  128/1 -> Magnitude Check/2
  64/1 -> XY Check/2
  32/1 -> Overflow/2
  4/1 -> Voltage Fault/2
  Logical Operator1/1 -> Subsystem1/1(Test_Lgc)
  MotAg1SyncErr/1 -> Logical Operator1/2, Boolean to uint8/1(InputBoolean)
  6372/1 -> Faults/2
  Compare To Zero6/1 -> Logical Operator1/1
  Boolean to u8/1(OutputNumber) -> Subsystem1/3(MotAg1NoAg)
  Boolean to uint8/1(OutputNumber) -> Subsystem1/2(MotAg1SyncErr)
  Subsystem1/1(ParamByte) -> ParamByte/1
  Magnitude Check/1 -> Compare To Zero2/1
  Compare To Zero/1 -> Boolean to u8/1(InputBoolean)
  Faults/1 -> Compare To Zero6/1
  "Boolean to u8     "/1(OutputNumber) -> Subsystem1/8(MotAg1VltgFlt)
  "Boolean to u8    "/1(OutputNumber) -> Subsystem1/7(MotAg1DSPOverFlow)
  "Boolean to u8 "/1(OutputNumber) -> Subsystem1/4(MotAg1NoXY)
  "Boolean to u8  "/1(OutputNumber) -> Subsystem1/5(MotAg1OutofLim)
  "Boolean to u8   "/1(OutputNumber) -> Subsystem1/6(MotAg1XYOutofLim)
  Compare To Zero1/1 -> "Boolean to u8 "/1(InputBoolean)
  Compare To Zero5/1 -> "Boolean to u8     "/1(InputBoolean)
  Compare To Zero4/1 -> "Boolean to u8    "/1(InputBoolean)
  No Valid XY/1 -> Compare To Zero1/1
  Compare To Zero2/1 -> "Boolean to u8  "/1(InputBoolean)
  Compare To Zero3/1 -> "Boolean to u8   "/1(InputBoolean)
  XY Check/1 -> Compare To Zero3/1
  Overflow/1 -> Compare To Zero4/1
  Voltage Fault/1 -> Compare To Zero5/1
  No GMR Angle/1 -> Compare To Zero/1
  MotAg1StatReg/1 -> No GMR Angle/1, No Valid XY/1, Magnitude Check/1, XY Check/1, Voltage Fault/1, Overflow/1, Faults/1

== system CM640C_MotAg1Meas/MotAg1Meas/MotAg1MeasPer2/MotAg1Calcn/MotAg1Processing/Offset Compensation /CopyRight2 ==

== system CM640C_MotAg1Meas/MotAg1Meas/MotAg1MeasPer2/MotAg1Calcn/MotAg1Processing/Offset Compensation /First Time Offset Calcn ==
  MotAg4Mecl : Inport  RequirementInfo={} %GIDa_25aaecee_4f2e_400f_abc5_f2372d041e99
  MotAg1SpiMecl : Inport  RequirementInfo={} %GIDa_27418f5d_8a5b_4847_ba52_ca2cb341472d  Port=2
  Action Port : ActionPort  ActionType=then
  Constant : Constant  OutDataTypeStr=uint8
  CopyRight2 : Subsystem  Description=|  mask(Copyright Information){none=on}
      | Copyright info block.                                               
      |                                                                     
      | Place copyright information at the top of every subsystem in design.
      mask prompts: none "No parameters"
      mask help: Place copyright information at the top of every subsystem in design.
      mask Display:
      | NxtrConf = 'Nexteer Confidential';
      | 
      | sys = bdroot; %handle for the current model ("system")
      | first = get_param(sys,'Created');
      | first = first(end-3:end);  %year is last four digits
      | 
      | last = get_param(sys,'LastModifiedDate');
      | if isempty(last)
      |     last = datestr(now,'yyyy');
      | else
      |     last = last(end-3:end);
      | end
      | 
      | if strcmp(first,last)
      |     fprintf('%s -- Copyright %s Nexteer',NxtrConf,first)
      | else
      |     fprintf('%s -- %s%s- %s Nexteer',NxtrConf,char(169),first,last)
      | end
  Data Store Read : DataStoreRead  DataStoreName=MotAg1InitOffs
  Data Store Write : DataStoreWrite  DataStoreName=MotAg1InitOffs
  Data Type Conversion : DataTypeConversion  OutDataTypeStr=int32
  Data Type Conversion1 : DataTypeConversion  OutDataTypeStr=int32
  Subtract : Sum  Inputs=+-
  Subtract1 : Sum
  MotAg1Offs : Outport
  wires:
  MotAg1SpiMecl/1 -> Data Type Conversion1/1
  Data Type Conversion/1 -> Subtract/1
  Data Type Conversion1/1 -> Subtract/2
  MotAg4Mecl/1 -> Data Type Conversion/1
  Constant/1 -> Subtract1/2
  Subtract1/1 -> Data Store Write/1
  Data Store Read/1 -> Subtract1/1
  Subtract/1 -> MotAg1Offs/1

== system CM640C_MotAg1Meas/MotAg1Meas/MotAg1MeasPer2/MotAg1Calcn/MotAg1Processing/Offset Compensation /Rt Offs Calcn ==
  MotAg4Mecl : Inport  RequirementInfo={} %GIDa_68f0f226_5b53_4cfc_a377_050a14e64919
  MotAg1SpiMecl : Inport  RequirementInfo={} %GIDa_5deca769_324c_4965_b2f5_c5a430060931  Port=2
  Action Port : ActionPort  ActionType=else
  CopyRight2 : Subsystem  Description=|  mask(Copyright Information){none=on}
      | Copyright info block.                                               
      |                                                                     
      | Place copyright information at the top of every subsystem in design.
      mask prompts: none "No parameters"
      mask help: Place copyright information at the top of every subsystem in design.
      mask Display:
      | NxtrConf = 'Nexteer Confidential';
      | 
      | sys = bdroot; %handle for the current model ("system")
      | first = get_param(sys,'Created');
      | first = first(end-3:end);  %year is last four digits
      | 
      | last = get_param(sys,'LastModifiedDate');
      | if isempty(last)
      |     last = datestr(now,'yyyy');
      | else
      |     last = last(end-3:end);
      | end
      | 
      | if strcmp(first,last)
      |     fprintf('%s -- Copyright %s Nexteer',NxtrConf,first)
      | else
      |     fprintf('%s -- %s%s- %s Nexteer',NxtrConf,char(169),first,last)
      | end
  Data Store Read1 : DataStoreRead  DataStoreName=MotAg1PrevOffs
  Data Type Conversion : DataTypeConversion  OutDataTypeStr=int32
  Data Type Conversion1 : DataTypeConversion  OutDataTypeStr=int32
  Subtract : Sum  Inputs=+-
  MotAg1Offs : Outport
  MotAg1RtOffs : Outport  Port=2
  wires:
  MotAg4Mecl/1 -> Data Type Conversion/1
  Subtract/1 -> MotAg1RtOffs/1
  Data Type Conversion1/1 -> Subtract/2
  Data Type Conversion/1 -> Subtract/1
  MotAg1SpiMecl/1 -> Data Type Conversion1/1
  Data Store Read1/1 -> MotAg1Offs/1

== system CM640C_MotAg1Meas/MotAg1Meas/MotAg1MeasPer2/MotAg1Calcn/MotAg1Processing/SPI  Motor Angle Calcn/CopyRight1 ==

== system CM640C_MotAg1Meas/MotAg1Meas/MotAg1MeasPer2/MotAg1Calcn/MotAg1Processing/SPI  Motor Angle Calcn/Polarity Correction ==
  MotAg1RawSpiMecl : Inport
  MotAgMecl1Polarity : Inport  Port=2
  CopyRight1 : Subsystem  Description=|  mask(Copyright Information){none=on}
      | Copyright info block.                                               
      |                                                                     
      | Place copyright information at the top of every subsystem in design.
      mask prompts: none "No parameters"
      mask help: Place copyright information at the top of every subsystem in design.
      mask Display:
      | NxtrConf = 'Nexteer Confidential';
      | 
      | sys = bdroot; %handle for the current model ("system")
      | first = get_param(sys,'Created');
      | first = first(end-3:end);  %year is last four digits
      | 
      | last = get_param(sys,'LastModifiedDate');
      | if isempty(last)
      |     last = datestr(now,'yyyy');
      | else
      |     last = last(end-3:end);
      | end
      | 
      | if strcmp(first,last)
      |     fprintf('%s -- Copyright %s Nexteer',NxtrConf,first)
      | else
      |     fprintf('%s -- %s%s- %s Nexteer',NxtrConf,char(169),first,last)
      | end
  Data Store Write : DataStoreWrite  DataStoreName=dMotAg1MeasMotAg1SpiMecl
  If : If  IfExpression=u1 < 0
  Merge : Merge
  Negative Polarity : Subsystem  TreatAsAtomicUnit=on
  Positive Polarity : Subsystem  TreatAsAtomicUnit=on
  MotAg1SpiMecl : Outport
  wires:
  MotAgMecl1Polarity/1 -> If/1
  MotAg1RawSpiMecl/1 -> Negative Polarity/1(MotAg1RawSpiMecl), Positive Polarity/1(MotAg1RawSpiMecl)
  If/1 -> Negative Polarity/Action
  If/2 -> Positive Polarity/Action
  Negative Polarity/1(MotAg1SpiPolarityCorrd) -> Merge/1
  Positive Polarity/1(MotAg1SpiPolarityCorrd) -> Merge/2
  Merge/1 -> MotAg1SpiMecl/1, Data Store Write/1

== system CM640C_MotAg1Meas/MotAg1Meas/MotAg1MeasPer2/MotAg1Calcn/MotAg1Processing/SPI IIF Motor Angle/CopyRight2 ==
